simulink model "SwarmDroneCounterSHI"  (R2025b)
settings: Solver=VariableStepAuto  StartTime=0.0  StopTime=50.0  RelTol=1e-3
libraries: simulink x1
settings Model: Creator=PRANAV  LastModifiedBy=PRANAV

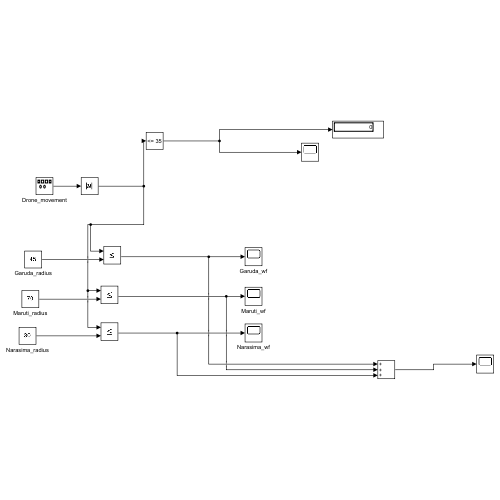
[thumbnail: Simulink's stored preview of the top-level diagram]
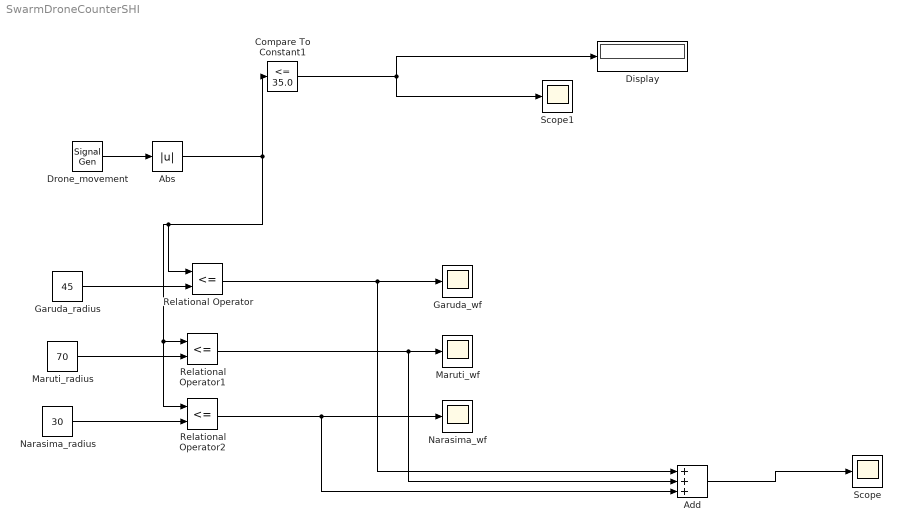
== system SwarmDroneCounterSHI ==
  Abs : Abs  SaturateOnIntegerOverflow=off
  Add : Sum  Inputs=+++
  Compare To Constant1 : simulink/Logic and Bit Operations/Compare To Constant  relop=<=  const=35.0  OutDataTypeStr=boolean
  Display : Display
  Drone_movement : SignalGenerator  Amplitude=150  Frequency=0.2  Units=rad/sec
  Garuda_radius : Constant  Value=45
  Garuda_wf : Scope
      settings: ActiveDisplayYMinimum=-0.12499999999999997  ActiveDisplayYMaximum=1.125
  Maruti_radius : Constant  Value=70
  Maruti_wf : Scope
      settings: ActiveDisplayYMinimum=-0.12499999999999997  ActiveDisplayYMaximum=1.125  DataLoggingVariableName=ScopeData2
  Narasima_radius : Constant  Value=30
  Narasima_wf : Scope
      settings: ActiveDisplayYMinimum=-0.12499999999999997  ActiveDisplayYMaximum=1.125  DataLoggingVariableName=ScopeData3
  Relational Operator : RelationalOperator  Operator=<=  OutDataTypeStr=boolean  RndMeth=Simplest  InputSameDT=off
  Relational Operator1 : RelationalOperator  Operator=<=  OutDataTypeStr=boolean  RndMeth=Simplest  InputSameDT=off
  Relational Operator2 : RelationalOperator  Operator=<=  OutDataTypeStr=boolean  RndMeth=Simplest  InputSameDT=off
  Scope : Scope
      settings: ActiveDisplayYMinimum=-0.37499999999999989  ActiveDisplayYMaximum=3.375  DataLoggingVariableName=ScopeData4
  Scope1 : Scope
      settings: ActiveDisplayYMinimum=-1  ActiveDisplayYMaximum=1
  wires:
  Drone_movement/1 -> Abs/1
  Abs/1 -> Relational Operator2/1, Relational Operator1/1, Relational Operator/1, Compare To Constant1/1
  Compare To Constant1/1 -> Scope1/1, Display/1
  Garuda_radius/1 -> Relational Operator/2
  Maruti_radius/1 -> Relational Operator1/2
  Narasima_radius/1 -> Relational Operator2/2
  Relational Operator/1 -> Add/1, Garuda_wf/1
  Relational Operator1/1 -> Add/2, Maruti_wf/1
  Relational Operator2/1 -> Add/3, Narasima_wf/1
  Add/1 -> Scope/1
